simulink model "TST_T50_VD"  (R2016b)
settings: Solver=FixedStepDiscrete  StartTime=0.0  StopTime=simTime  FixedStep=sampleTime  RelTol=1e-3
values from neighbouring files (symbols this model uses):
  testCase = 1    [initTST_T50_VD_001.m]
libraries: UnitTest_Lib x3, simulink x2
settings Model: Creator=liangyunbo  LastModifiedBy=liangyunbo
settings DebuggingCC: SignalRangeChecking=error

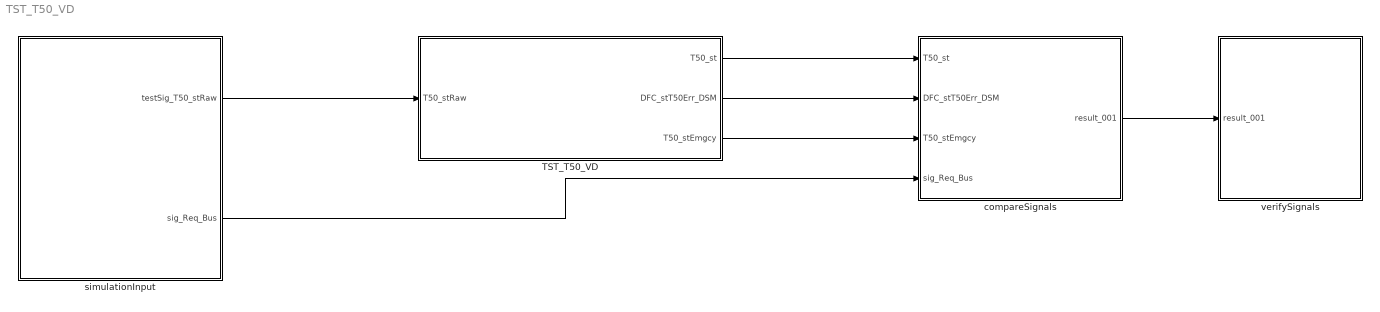
== system TST_T50_VD ==
  TST_T50_VD : Subsystem
  compareSignals : Subsystem
  simulationInput : Subsystem
  verifySignals : Subsystem
  wires:
  simulationInput/1(testSig_T50_stRaw) -> TST_T50_VD/1(T50_stRaw)
  TST_T50_VD/1(T50_st) -> compareSignals/1(T50_st)
  TST_T50_VD/2(DFC_stT50Err_DSM) -> compareSignals/2(DFC_stT50Err_DSM)
  TST_T50_VD/3(T50_stEmgcy) -> compareSignals/3(T50_stEmgcy)
  simulationInput/2(sig_Req_Bus) -> compareSignals/4(sig_Req_Bus)
  compareSignals/1(result_001) -> verifySignals/1(result_001)

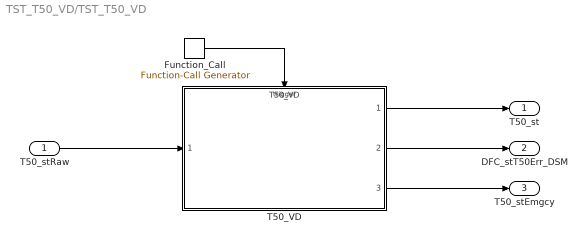
== system TST_T50_VD/TST_T50_VD ==
  T50_stRaw : Inport
  Function_Call : simulink/Ports & Subsystems/Function-Call Generator  sample_time=sampleTime  numberOfIterations=1
  T50_VD : ModelReference  ModelNameDialog=T50_VD  SimulationMode=Normal  ModelReferenceVersion=1.58  TriggerPortName=function  TriggerPortTriggerType=function-call  TriggerPortStatesWhenEnabling=held
  T50_st : Outport
  DFC_stT50Err_DSM : Outport  Port=2
  T50_stEmgcy : Outport  Port=3
  wires:
  Function_Call/1 -> T50_VD/Trigger
  T50_stRaw/1 -> T50_VD/1
  T50_VD/1 -> T50_st/1
  T50_VD/2 -> DFC_stT50Err_DSM/1
  T50_VD/3 -> T50_stEmgcy/1

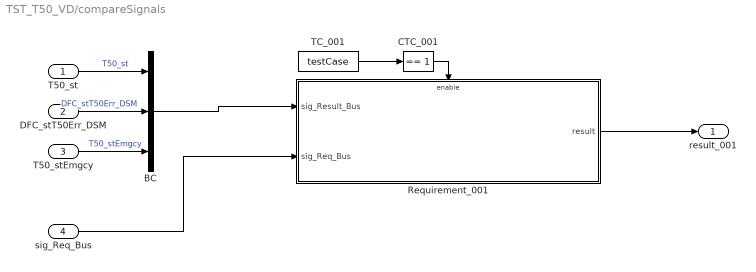
== system TST_T50_VD/compareSignals ==
  T50_st : Inport
  DFC_stT50Err_DSM : Inport  Port=2
  T50_stEmgcy : Inport  Port=3
  sig_Req_Bus : Inport  Port=4
  BC : BusCreator  Inputs=3
  CTC_001 : simulink/Logic and Bit Operations/Compare To Constant  relop===  const=1  OutDataTypeStr=boolean
  Requirement_001 : Subsystem
  TC_001 : Constant  Value=testCase
  result_001 : Outport
  wires:
  T50_st/1 -> BC/1  "T50_st"
  DFC_stT50Err_DSM/1 -> BC/2  "DFC_stT50Err_DSM"
  T50_stEmgcy/1 -> BC/3  "T50_stEmgcy"
  TC_001/1 -> CTC_001/1
  CTC_001/1 -> Requirement_001/Enable
  sig_Req_Bus/1 -> Requirement_001/2(sig_Req_Bus)
  BC/1 -> Requirement_001/1(sig_Result_Bus)
  Requirement_001/1(result) -> result_001/1

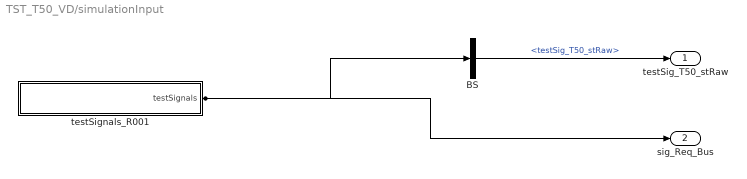
== system TST_T50_VD/simulationInput ==
  BS : BusSelector  OutputSignals=testSig_T50_stRaw
  testSignals_R001 : Subsystem
  testSig_T50_stRaw : Outport
  sig_Req_Bus : Outport  Port=2
  wires:
  BS/1 -> testSig_T50_stRaw/1  "<testSig_T50_stRaw>"
  testSignals_R001/1(testSignals) -> BS/1, sig_Req_Bus/1

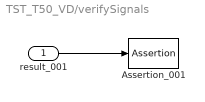
== system TST_T50_VD/verifySignals ==
  result_001 : Inport
  Assertion_001 : Assertion  Enabled=off
  wires:
  result_001/1 -> Assertion_001/1

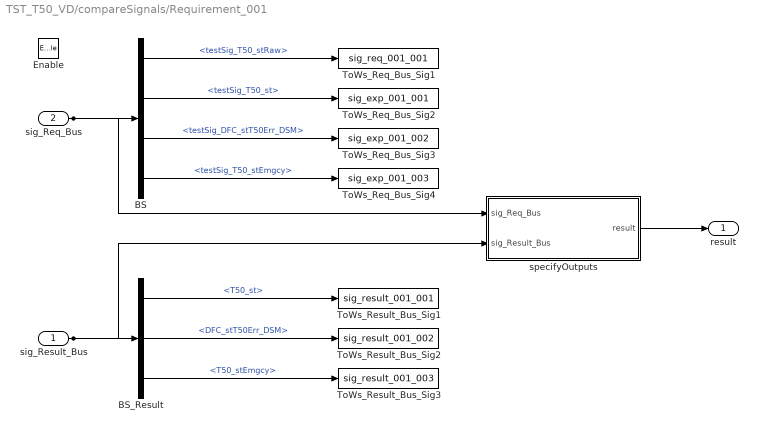
== system TST_T50_VD/compareSignals/Requirement_001 ==
  sig_Result_Bus : Inport
  sig_Req_Bus : Inport  Port=2
  Enable : EnablePort
  BS : BusSelector  OutputSignals=testSig_T50_stRaw,testSig_T50_st,testSig_DFC_stT50Err_DSM,testSig_T50_stEmgcy
  BS_Result : BusSelector  OutputSignals=T50_st,DFC_stT50Err_DSM,T50_stEmgcy
  ToWs_Req_Bus_Sig1 : ToWorkspace  VariableName=sig_req_001_001  SaveFormat=Structure With Time
  ToWs_Req_Bus_Sig2 : ToWorkspace  VariableName=sig_exp_001_001  SaveFormat=Structure With Time
  ToWs_Req_Bus_Sig3 : ToWorkspace  VariableName=sig_exp_001_002  SaveFormat=Structure With Time
  ToWs_Req_Bus_Sig4 : ToWorkspace  VariableName=sig_exp_001_003  SaveFormat=Structure With Time
  ToWs_Result_Bus_Sig1 : ToWorkspace  VariableName=sig_result_001_001  SaveFormat=Structure With Time
  ToWs_Result_Bus_Sig2 : ToWorkspace  VariableName=sig_result_001_002  SaveFormat=Structure With Time
  ToWs_Result_Bus_Sig3 : ToWorkspace  VariableName=sig_result_001_003  SaveFormat=Structure With Time
  specifyOutputs : Subsystem
  result : Outport
  wires:
  sig_Req_Bus/1 -> BS/1, specifyOutputs/1(sig_Req_Bus)
  BS/1 -> ToWs_Req_Bus_Sig1/1  "<testSig_T50_stRaw>"
  BS/2 -> ToWs_Req_Bus_Sig2/1  "<testSig_T50_st>"
  BS/3 -> ToWs_Req_Bus_Sig3/1  "<testSig_DFC_stT50Err_DSM>"
  BS/4 -> ToWs_Req_Bus_Sig4/1  "<testSig_T50_stEmgcy>"
  sig_Result_Bus/1 -> BS_Result/1, specifyOutputs/2(sig_Result_Bus)
  BS_Result/1 -> ToWs_Result_Bus_Sig1/1  "<T50_st>"
  BS_Result/2 -> ToWs_Result_Bus_Sig2/1  "<DFC_stT50Err_DSM>"
  BS_Result/3 -> ToWs_Result_Bus_Sig3/1  "<T50_stEmgcy>"
  specifyOutputs/1(result) -> result/1

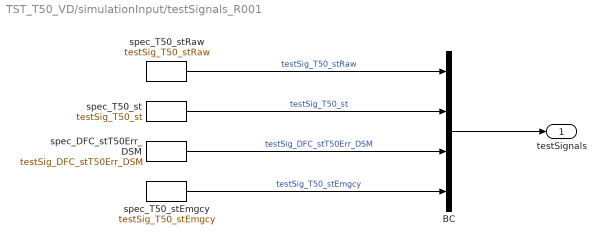
== system TST_T50_VD/simulationInput/testSignals_R001 ==
  BC : BusCreator  Inputs=4
  spec_DFC_stT50Err_DSM : FromWorkspace  VariableName=testSig_DFC_stT50Err_DSM  Interpolate=off  OutputAfterFinalValue=Holding final value
  spec_T50_st : FromWorkspace  VariableName=testSig_T50_st  Interpolate=off  OutputAfterFinalValue=Holding final value
  spec_T50_stEmgcy : FromWorkspace  VariableName=testSig_T50_stEmgcy  Interpolate=off  OutputAfterFinalValue=Holding final value
  spec_T50_stRaw : FromWorkspace  VariableName=testSig_T50_stRaw  Interpolate=off  OutputAfterFinalValue=Holding final value
  testSignals : Outport
  wires:
  BC/1 -> testSignals/1
  spec_T50_stRaw/1 -> BC/1  "testSig_T50_stRaw"
  spec_T50_st/1 -> BC/2  "testSig_T50_st"
  spec_DFC_stT50Err_DSM/1 -> BC/3  "testSig_DFC_stT50Err_DSM"
  spec_T50_stEmgcy/1 -> BC/4  "testSig_T50_stEmgcy"

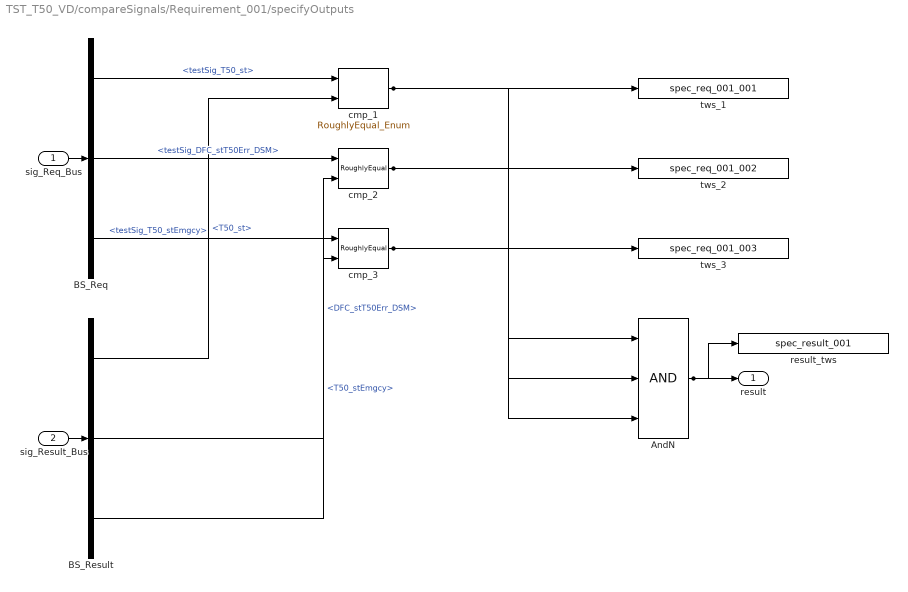
== system TST_T50_VD/compareSignals/Requirement_001/specifyOutputs ==
  sig_Req_Bus : Inport
  sig_Result_Bus : Inport  Port=2
  AndN : Logic  Inputs=3
  BS_Req : BusSelector  OutputSignals=testSig_T50_st,testSig_DFC_stT50Err_DSM,testSig_T50_stEmgcy
  BS_Result : BusSelector  OutputSignals=T50_st,DFC_stT50Err_DSM,T50_stEmgcy
  cmp_1 : UnitTest_Lib/RoughlyEqual_Enum  slope=0.1
  cmp_2 : UnitTest_Lib/RoughlyEqual  slope=0.1
  cmp_3 : UnitTest_Lib/RoughlyEqual  slope=0.1
  result_tws : ToWorkspace  VariableName=spec_result_001
  tws_1 : ToWorkspace  VariableName=spec_req_001_001
  tws_2 : ToWorkspace  VariableName=spec_req_001_002
  tws_3 : ToWorkspace  VariableName=spec_req_001_003
  result : Outport
  wires:
  sig_Req_Bus/1 -> BS_Req/1
  sig_Result_Bus/1 -> BS_Result/1
  AndN/1 -> result/1, result_tws/1
  BS_Req/1 -> cmp_1/1  "<testSig_T50_st>"
  BS_Result/1 -> cmp_1/2  "<T50_st>"
  cmp_1/1 -> tws_1/1, AndN/1
  BS_Req/2 -> cmp_2/1  "<testSig_DFC_stT50Err_DSM>"
  BS_Result/2 -> cmp_2/2  "<DFC_stT50Err_DSM>"
  cmp_2/1 -> tws_2/1, AndN/2
  BS_Req/3 -> cmp_3/1  "<testSig_T50_stEmgcy>"
  BS_Result/3 -> cmp_3/2  "<T50_stEmgcy>"
  cmp_3/1 -> tws_3/1, AndN/3
